simulink model "SimLin"  (R2024a)
settings: Solver=ode45  StartTime=0.0  StopTime=10.0  RelTol=1e-3  EnableMultiTasking=on
undefined symbols (not defined in the file or in its folder): ParamReels
settings Model: Creator=Nazih  LastModifiedBy=Administrator
settings SolverCC: AlgebraicLoopSolver=TrustRegion
settings DataIOCC: LimitDataPoints=on  SaveFormat=Array  SignalLoggingSaveFormat=ModelDataLogs  ReturnWorkspaceOutputs=off
settings OptimizationCC: BlockReduction=off  BooleanDataType=off  ExpressionDepthLimit=2147483647  InitFltsAndDblsToZero=on  LifeSpan=inf
settings DebuggingCC: SaveWithParameterizedLinksMsg=none  UnderspecifiedInitializationDetection=Classic  MergeDetectMultiDrivingBlocksExec=none  SignalResolutionControl=TryResolveAllWithWarning  MultiTaskDSMMsg=warning  MultiTaskCondExecSysMsg=none  FcnCallInpInsideContextMsg=warning  UnconnectedInputMsg=warning  UnconnectedOutputMsg=warning  UnconnectedLineMsg=warning  StateNameClashWarn=warning  SFUnexpectedBacktrackingDiag=warning  SFNoUnconditionalDefaultTransitionDiag=warning  SFExecutionAtInitializationDiag=none  ArithmeticOperatorsInVariantConditions=warning
settings HardwareCC: ProdBitPerPointer=32  ProdBitPerSizeT=32  ProdBitPerPtrDiffT=32  ProdLargestAtomicFloat=None  ProdIntDivRoundTo=Undefined  ProdEndianess=Unspecified  ProdWordSize=32  ProdHWDeviceType=32-bit Generic  TargetUnknown=on
settings ModelReferenceCC: PropagateSignalLabelsOutOfModel=off
settings SFSimCC: SimUseLocalCustomCode=off  CustomCodeUndefinedFunction=UseInterfaceOnly
settings RTWCC: RTWUseLocalCustomCode=off  GPUComputeCapability=3.5
settings CodeAppCC: StateflowObjectComments=on
settings GRTTargetCC: TargetFcnLib=ansi_tfl_tmw.mat  TargetLangStandard=C89/C90 (ANSI)  CombineOutputUpdateFcns=off  GRTInterface=on
settings ConfigComp: CovMetricSettings=dw  CovSaveCumulativeToWorkspaceVar=on  CovSaveSingleToWorkspaceVar=on  CovExternalEMLEnable=off

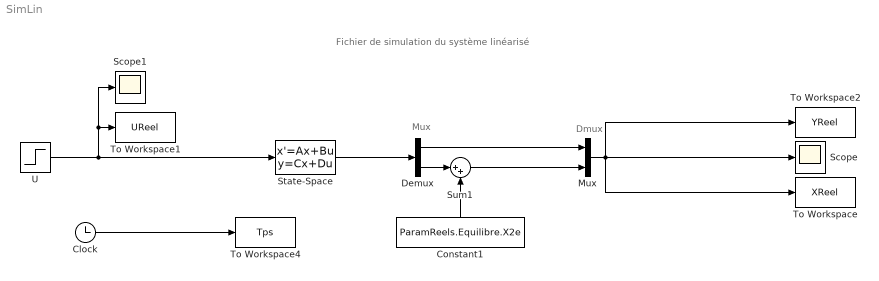
== system SimLin ==
  note: Fichier de simulation du système linéarisé
  note: Mux
  note: Dmux
  Clock : Clock
  Constant1 : Constant  Value=ParamReels.Equilibre.X2e
  Demux : Demux  Outputs=2
      settings: DisplayOption=none
  Mux : Mux  Inputs=2
  Scope : Scope
  Scope1 : Scope
  State-Space : StateSpace  A=ParamReels.A  B=ParamReels.B  C=eye(2)  D=zeros(2,1)  InitialCondition=ParamReels.X0lin
  Sum1 : Sum  Inputs=|++  InputSameDT=on  SaturateOnIntegerOverflow=on  OutDataTypeStr=Inherit: Same as first input
  To Workspace : ToWorkspace  VariableName=XReel  SampleTime=ParamReels.Te
  To Workspace1 : ToWorkspace  VariableName=UReel  SampleTime=ParamReels.Te
  To Workspace2 : ToWorkspace  VariableName=YReel  SampleTime=ParamReels.Te
  To Workspace4 : ToWorkspace  VariableName=Tps  SampleTime=ParamReels.Te
  U : Step  Time=4  Before=ParamReels.Equilibre.Ue  After=ParamReels.Equilibre.Ue + 1  SampleTime=0
  wires:
  State-Space/1 -> Demux/1
  Demux/2 -> Sum1/1
  Constant1/1 -> Sum1/2
  Sum1/1 -> Mux/2
  Demux/1 -> Mux/1
  Mux/1 -> To Workspace2/1, Scope/1, To Workspace/1
  Clock/1 -> To Workspace4/1
  U/1 -> To Workspace1/1, Scope1/1, State-Space/1
